simulink model "vcu"  (R2024b)
settings: Solver=FixedStepAuto  StartTime=0.0  StopTime=2000  FixedStep=0.001  RelTol=1e-3
libraries: canoelib x9
settings Model: Creator=USER  LastModifiedBy=USER
settings DebuggingCC: AlgebraicLoopMsg=none

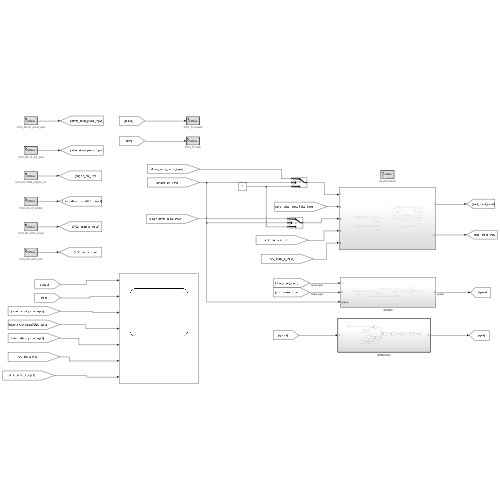
[thumbnail: Simulink's stored preview of the top-level diagram]
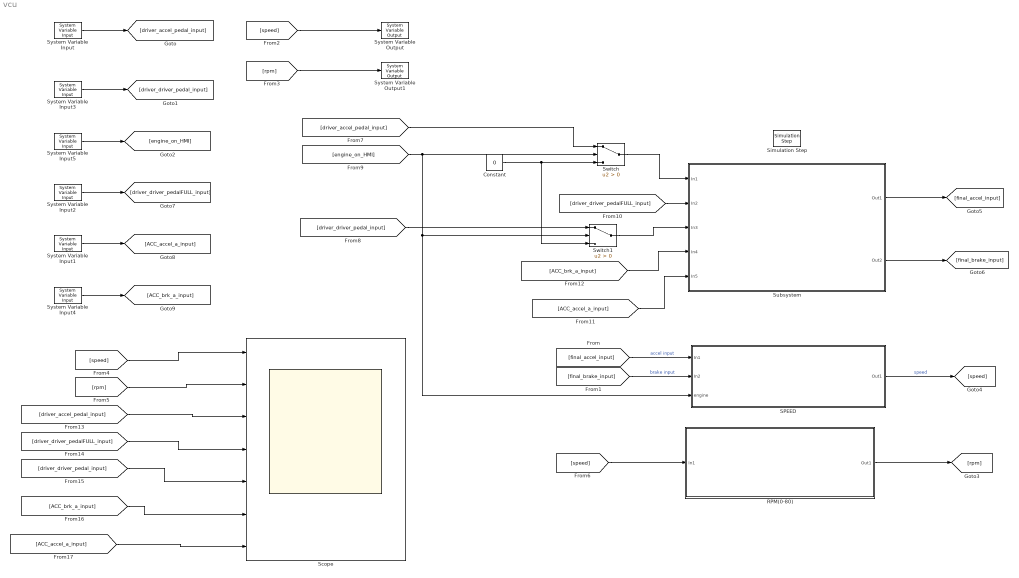
== system vcu ==
  Constant : Constant  Value=0
  RPM(0-80) : Subsystem  TreatAsAtomicUnit=on  SystemSampleTime=1
  SPEED : Subsystem
  Scope : Scope  NumInputPorts=7
  Simulation Step : canoelib/CANoe I//O/Simulation Step  mode=Synchronized
      settings: AttributesFormatString=%<mode>  SourceProductName=Vector CANoe
  Subsystem : Subsystem
  Switch : Switch  Criteria=u2 > Threshold  SaturateOnIntegerOverflow=off  InputSameDT=off
  Switch1 : Switch  Criteria=u2 > Threshold  SaturateOnIntegerOverflow=off  InputSameDT=off
  System Variable Input : canoelib/CANoe I//O/System Variable Input  nsName=VCU_Rx  sysVarName=dr_accel_ped  arrayIndex=-1  editSampleTime=0  rawValue=Default  dataType=Default  dataTypeDB=int32  hasEncoding=off  dataTypeCANoe=Get from CANoe
      settings: AttributesFormatString=%<nsName>::%<sysVarName>  SourceProductName=Vector CANoe
  System Variable Input1 : canoelib/CANoe I//O/System Variable Input  nsName=VCU_Rx  sysVarName=ACC_accel  arrayIndex=-1  editSampleTime=0  rawValue=Default  dataType=Default  dataTypeDB=int32  hasEncoding=off  dataTypeCANoe=Get from CANoe
      settings: AttributesFormatString=%<nsName>::%<sysVarName>  SourceProductName=Vector CANoe
  System Variable Input2 : canoelib/CANoe I//O/System Variable Input  nsName=VCU_Rx  sysVarName=dr_brkfull  arrayIndex=-1  editSampleTime=0  rawValue=Default  dataType=Default  dataTypeDB=int32  hasEncoding=off  dataTypeCANoe=Get from CANoe
      settings: AttributesFormatString=%<nsName>::%<sysVarName>  SourceProductName=Vector CANoe
  System Variable Input3 : canoelib/CANoe I//O/System Variable Input  nsName=VCU_Rx  sysVarName=dr_brk_ped  arrayIndex=-1  editSampleTime=0  rawValue=Default  dataType=Default  dataTypeDB=int32  hasEncoding=off  dataTypeCANoe=Get from CANoe
      settings: AttributesFormatString=%<nsName>::%<sysVarName>  SourceProductName=Vector CANoe
  System Variable Input4 : canoelib/CANoe I//O/System Variable Input  nsName=VCU_Rx  sysVarName=ACC_brk  arrayIndex=-1  editSampleTime=0  rawValue=Default  dataType=Default  dataTypeDB=int32  hasEncoding=off  dataTypeCANoe=Get from CANoe
      settings: AttributesFormatString=%<nsName>::%<sysVarName>  SourceProductName=Vector CANoe
  System Variable Input5 : canoelib/CANoe I//O/System Variable Input  nsName=VCU_Rx  sysVarName=HMI_engine_on  arrayIndex=-1  editSampleTime=0  rawValue=Default  dataType=Default  dataTypeDB=int32  hasEncoding=off  dataTypeCANoe=Get from CANoe
      settings: AttributesFormatString=%<nsName>::%<sysVarName>  SourceProductName=Vector CANoe
  System Variable Output : canoelib/CANoe I//O/System Variable Output  nsName=VCU_Tx  sysVarName=speed  arrayIndex=-1  rawValue=Default  dataType=Default  dataTypeDB=int32  hasEncoding=off  dataTypeCANoe=Get from CANoe
      settings: AttributesFormatString=%<nsName>::%<sysVarName>  SourceProductName=Vector CANoe
  System Variable Output1 : canoelib/CANoe I//O/System Variable Output  nsName=VCU_Tx  sysVarName=rpm  arrayIndex=-1  rawValue=Default  dataType=Default  dataTypeDB=int32  hasEncoding=off  dataTypeCANoe=Get from CANoe
      settings: AttributesFormatString=%<nsName>::%<sysVarName>  SourceProductName=Vector CANoe
  wires:
  [rpm] -> System Variable Output1/1
  [final_accel_input] -> SPEED/1(In1)  "accel input"
  [final_brake_input] -> SPEED/2(In2)  "brake input"
  SPEED/1(Out1) -> [speed]  "speed"
  [speed] -> RPM(0-80)/1(In1)
  RPM(0-80)/1(Out1) -> [rpm]
  Switch/1 -> Subsystem/1(In1)
  Constant/1 -> Switch1/3, Switch/3
  Switch1/1 -> Subsystem/3(In3)
  Subsystem/2(Out2) -> [final_brake_input]
  Subsystem/1(Out1) -> [final_accel_input]
  [speed] -> Scope/1
  [rpm] -> Scope/2
  System Variable Input/1 -> [driver_accel_pedal_input]
  System Variable Input3/1 -> [driver_driver_pedal_input]
  [driver_accel_pedal_input] -> Switch/1
  [driver_driver_pedal_input] -> Switch1/1
  System Variable Input5/1 -> [engine_on_HMI]
  [engine_on_HMI] -> SPEED/3(engine), Switch1/2, Switch/2
  [driver_driver_pedalFULL_input] -> Subsystem/2(In2)
  System Variable Input2/1 -> [driver_driver_pedalFULL_input]
  System Variable Input1/1 -> [ACC_accel_a_input]
  [ACC_accel_a_input] -> Subsystem/5(In5)
  System Variable Input4/1 -> [ACC_brk_a_input]
  [ACC_brk_a_input] -> Subsystem/4(In4)
  [speed] -> System Variable Output/1
  [driver_accel_pedal_input] -> Scope/3
  [driver_driver_pedalFULL_input] -> Scope/4
  [driver_driver_pedal_input] -> Scope/5
  [ACC_brk_a_input] -> Scope/6
  [ACC_accel_a_input] -> Scope/7

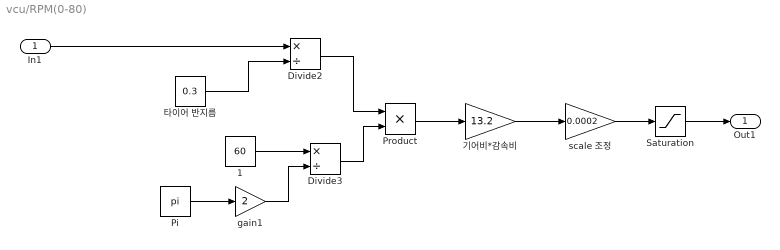
== system vcu/RPM(0-80) ==
  In1 : Inport
  " 1" : Constant  Value=60
  Divide2 : Product  Inputs=*/
  Divide3 : Product  Inputs=*/
  Pi : Constant  Value=pi  OutDataTypeStr=Inherit: Inherit via back propagation
  Product : Product
  Saturation : Saturate  UpperLimit=8  LowerLimit=1
  gain1 : Gain  Gain=2
  scale 조정 : Gain  Gain=0.0002
  기어비*감속비 : Gain  Gain=13.2
  타이어 반지름 : Constant  Value=0.3
  Out1 : Outport
  wires:
  기어비*감속비/1 -> scale 조정/1
  " 1"/1 -> Divide3/1
  Pi/1 -> gain1/1
  Divide3/1 -> Product/2
  Divide2/1 -> Product/1
  gain1/1 -> Divide3/2
  타이어 반지름/1 -> Divide2/2
  Product/1 -> 기어비*감속비/1
  In1/1 -> Divide2/1
  scale 조정/1 -> Saturation/1
  Saturation/1 -> Out1/1

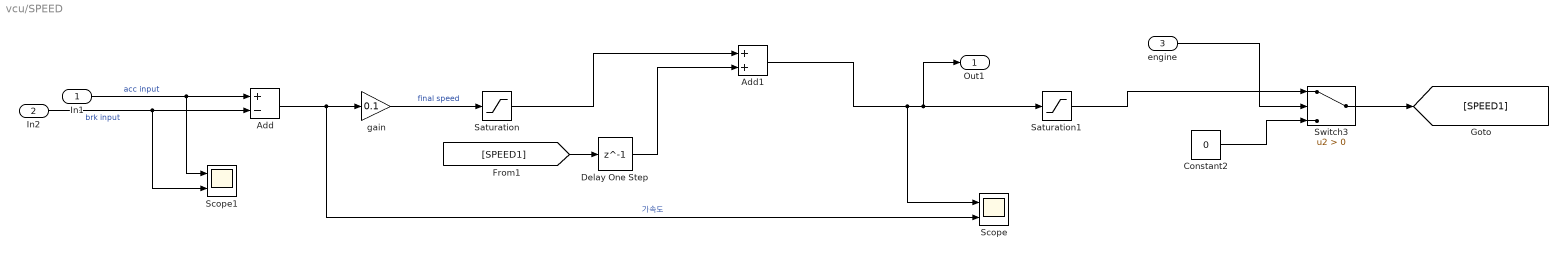
== system vcu/SPEED ==
  In1 : Inport
  In2 : Inport  Port=2
  engine : Inport  Port=3
  Add : Sum  Inputs=+-
  Add1 : Sum
  Constant2 : Constant  Value=0
  Delay One Step : Delay  DelayLength=1
  Saturation : Saturate  UpperLimit=10  LowerLimit=-5
  Saturation1 : Saturate  UpperLimit=280  LowerLimit=0
  Scope : Scope  NumInputPorts=2
  Scope1 : Scope  NumInputPorts=2
  Switch3 : Switch  Criteria=u2 > Threshold  SaturateOnIntegerOverflow=off  InputSameDT=off
  gain : Gain  Gain=0.1
  Out1 : Outport
  wires:
  In2/1 -> Scope1/2, Add/2  "brk input"
  Add/1 -> Scope/2, gain/1  "가속도"
  Saturation/1 -> Add1/1
  gain/1 -> Saturation/1  "final speed"
  In1/1 -> Add/1, Scope1/1  "acc input"
  [SPEED1] -> Delay One Step/1
  Delay One Step/1 -> Add1/2
  Add1/1 -> Scope/1, Out1/1, Saturation1/1
  engine/1 -> Switch3/2
  Saturation1/1 -> Switch3/1
  Constant2/1 -> Switch3/3
  Switch3/1 -> [SPEED1]

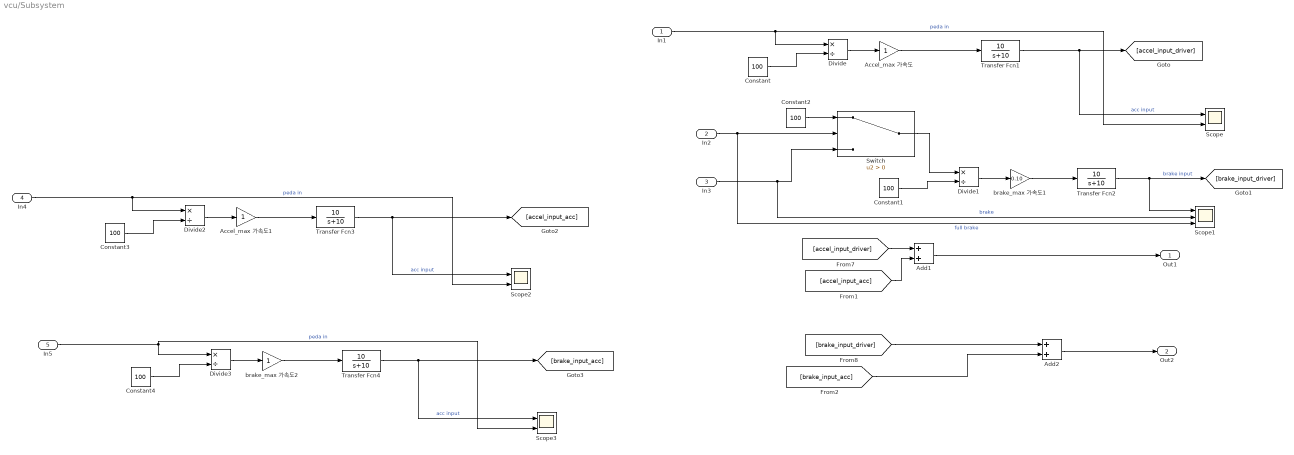
== system vcu/Subsystem ==
  In1 : Inport
  In2 : Inport  Port=2
  In3 : Inport  Port=3
  In4 : Inport  Port=4
  In5 : Inport  Port=5
  Accel_max 가속도 : Gain
  Accel_max 가속도1 : Gain
  Add1 : Sum
  Add2 : Sum
  Constant{,1..4} (5 alike) : Constant  Value=100
  Divide{,1..3} (4 alike) : Product  Inputs=*/
  Scope : Scope  NumInputPorts=2
  Scope1 : Scope  NumInputPorts=3
  Scope2 : Scope  NumInputPorts=2
  Scope3 : Scope  NumInputPorts=2
  Switch : Switch  Criteria=u2 > Threshold  SaturateOnIntegerOverflow=off  InputSameDT=off
  Transfer Fcn{1..4} (4 alike) : TransferFcn  Numerator=[10]  Denominator=[1 10]
  brake_max 가속도1 : Gain  Gain=0.10
  brake_max 가속도2 : Gain
  Out1 : Outport
  Out2 : Outport  Port=2
  wires:
  Constant/1 -> Divide/2
  Constant1/1 -> Divide1/2
  [accel_input_driver] -> Add1/1
  [brake_input_driver] -> Add2/1
  In2/1 -> Scope1/3, Switch/2  "full brake"
  brake_max 가속도1/1 -> Transfer Fcn2/1
  Divide/1 -> Accel_max 가속도/1
  Add2/1 -> Out2/1
  Divide1/1 -> brake_max 가속도1/1
  Switch/1 -> Divide1/1
  Constant2/1 -> Switch/1
  In1/1 -> Scope/2, Divide/1  "peda in"
  Add1/1 -> Out1/1
  In3/1 -> Scope1/2, Switch/3  "brake"
  Transfer Fcn1/1 -> Scope/1, [accel_input_driver]  "acc input"
  Transfer Fcn2/1 -> Scope1/1, [brake_input_driver]  "brake input"
  Accel_max 가속도/1 -> Transfer Fcn1/1
  Accel_max 가속도1/1 -> Transfer Fcn3/1
  Transfer Fcn3/1 -> Scope2/1, [accel_input_acc]  "acc input"
  In4/1 -> Scope2/2, Divide2/1  "peda in"
  Constant3/1 -> Divide2/2
  Divide2/1 -> Accel_max 가속도1/1
  [accel_input_acc] -> Add1/2
  In5/1 -> Scope3/2, Divide3/1  "peda in"
  Divide3/1 -> brake_max 가속도2/1
  Constant4/1 -> Divide3/2
  brake_max 가속도2/1 -> Transfer Fcn4/1
  Transfer Fcn4/1 -> Scope3/1, [brake_input_acc]  "acc input"
  [brake_input_acc] -> Add2/2
